simulink model "gyroModel"  (R2019b)
settings: Solver=VariableStepAuto  StartTime=0.0  StopTime=99.7  RelTol=1e-3
values from neighbouring files (symbols this model uses):
  bias = -0.85    [gyroParameters.m]
  w = 12.5*2*pi    (= 78.5398163397)    [gyroParameters.m]
  wn = 1000*2*pi    (= 6283.18530718)    [gyroParameters.m]
  z = zeta    [gyroParameters.m]
  zeta = sqrt(2)/2    [gyroParameters.m]
libraries: simulink x1
settings Model: OrderedModelArguments=off  Creator=covasanvictor  LastModifiedBy=covasanvictor

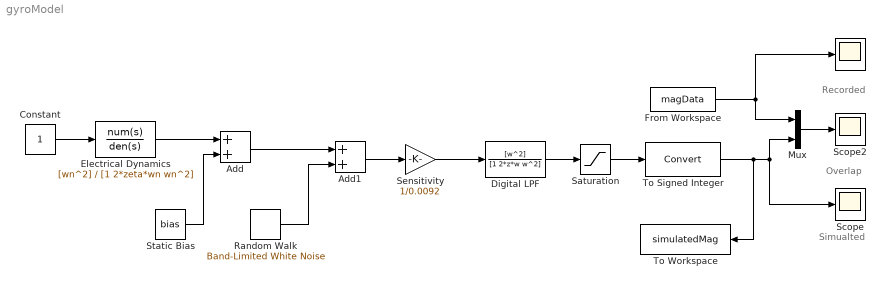
== system gyroModel ==
  note: Recorded
  note: Simualted
  note: Overlap
  " " : Scope
  Add : Sum
  Add1 : Sum
  Constant : Constant
  Digital LPF : TransferFcn  Numerator=[w^2]  Denominator=[1 2*z*w w^2]
  Electrical Dynamics : TransferFcn  Numerator=[wn^2]  Denominator=[1 2*zeta*wn wn^2]
  From Workspace : FromWorkspace  VariableName=magData  SampleTime=0
  Mux : Mux  Inputs=2
  "Random Walk " : simulink/Sources/Band-Limited White Noise  Cov=[power^2]  Ts=0.01  seed=[23341]
  Saturation : Saturate  UpperLimit=2^15  LowerLimit=-2^15
  Scope : Scope
  Scope2 : Scope
  Sensitivity : Gain  Gain=1/0.0092
  Static Bias : Constant  Value=bias
  To Signed Integer : DataTypeConversion
  To Workspace : ToWorkspace  VariableName=simulatedMag  SaveFormat=Timeseries  SampleTime=-1
  wires:
  Electrical Dynamics/1 -> Add/1
  Static Bias/1 -> Add/2
  "Random Walk "/1 -> Add1/2
  Add/1 -> Add1/1
  Add1/1 -> Sensitivity/1
  To Signed Integer/1 -> To Workspace/1, Mux/2, Scope/1
  Constant/1 -> Electrical Dynamics/1
  Sensitivity/1 -> Digital LPF/1
  Digital LPF/1 -> Saturation/1
  Saturation/1 -> To Signed Integer/1
  From Workspace/1 -> Mux/1, " "/1
  Mux/1 -> Scope2/1
